simulink model "02_Goniodsky_Mistry_EE547_Project"  (R2018b)
settings: Solver=FixedStepDiscrete  StartTime=0.0  StopTime=inf  RelTol=1e-3  EnableMultiTasking=on
undefined symbols (not defined in the file): DiscIntNeverNeededParam, K, rw
libraries: dspstat3 x2, arduinolib x1, dspsigops x1
settings Model: SimulationMode=external  ExtModeTrigDuration=2  Creator=gonio  LastModifiedBy=GAJJAR
settings OptimizationCC: EnhancedBackFolding=on  PassReuseOutputArgsAs=Individual arguments  MaxStackSize=64  OptimizeBlockOrder=speed  DifferentSizesBufferReuse=on  OptimizationCustomize=off
settings DebuggingCC: ParameterTunabilityLossMsg=error
settings HardwareCC: ProdBitPerInt=16  ProdBitPerPointer=16  ProdBitPerSizeT=16  ProdBitPerPtrDiffT=16  ProdLargestAtomicFloat=None  ProdWordSize=8  ProdHWDeviceType=Atmel->AVR  UseEmbeddedCoderFeatures=off  UseSimulinkCoderFeatures=off
settings SFSimCC: MATLABDynamicMemAlloc=off
settings RTWCC: SystemTargetFile=ert.tlc  HardwareBoard=Arduino Mega 2560  TemplateMakefile=ert_default_tmf  RTWVerbose=off  Toolchain=Arduino AVR  BuildConfiguration=Faster Runs  IncludeHyperlinkInReport=on
settings CodeAppCC: ForceParamTrailComments=on  OperatorAnnotations=on  SimulinkDataObjDesc=on  SFDataObjDesc=on  MangleLength=10  InsertBlockDesc=on
settings ERTTargetCC: SupportContinuousTime=on  SupportNonInlinedSFcns=on  SupportVariableSizeSignals=on  ExtMode=on  ExtModeMexArgs='127.0.0.1' 0 17725  ERTSrcFileBannerTemplate=codertarget_code_template.cgt  ERTHdrFileBannerTemplate=codertarget_code_template.cgt  ERTDataSrcFileTemplate=codertarget_code_template.cgt  ERTDataHdrFileTemplate=codertarget_code_template.cgt

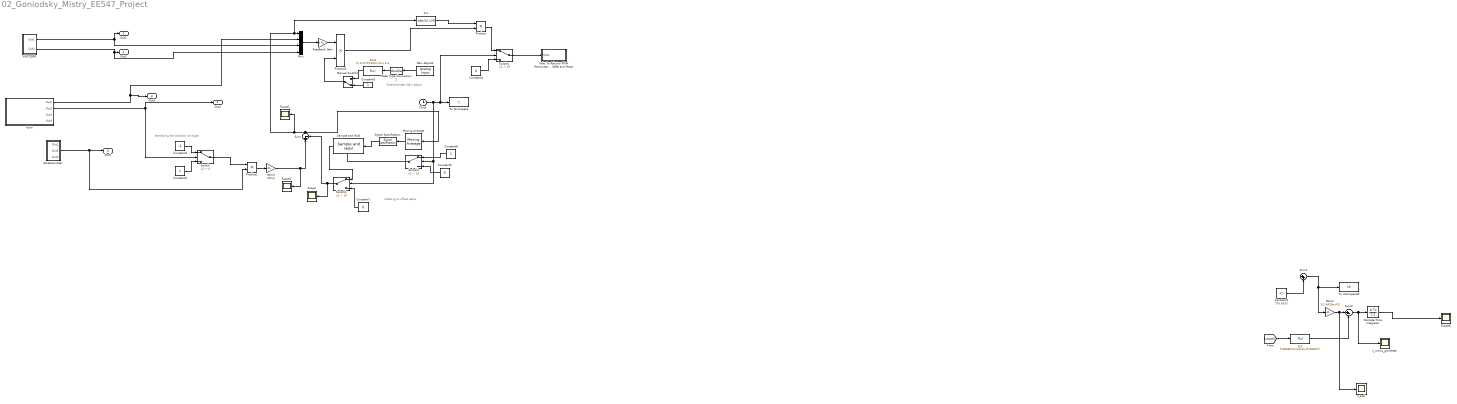
== system 02_Goniodsky_Mistry_EE547_Project ==
  note: Potentiometer Gain Adjust
  note: Identifying the Direction of angle
  note: Intitial gyro offset setup
  Accelerometer : Subsystem
  Clock : Clock
  Constant1 : Constant  Value=376.6633
  Constant2 : Constant
  Constant3 : Constant  Value=-1
  Constant4 : Constant  Value=0
  Constant5 : Constant  Value=0
  Constant6 : Constant
  Constant7 : Constant  Value=0
  Constant9 : Constant
  Data Type Conversion1 : DataTypeConversion  OutDataTypeStr=double
  Discrete-Time Integrator : DiscreteIntegrator  SampleTime=-1  ICPrevOutput=DiscIntNeverNeededParam  ICPrevScaledInput=DiscIntNeverNeededParam
  "ENCODER " : Subsystem
  Fcn : Fcn  Expr=abs(u)<20
  Fcn2 : Fcn  Expr=(1-1/4)*2/1023*u(1)+1/4
  Feedback Gain : Gain  Gain=K  Multiplication=Matrix(K*u)
  Gain Adjust2 : arduinolib/Analog Input  pinNumber=0  ReadResultsOnly=off  ConversionTriggerSource=Software  ExternalTriggerType=uint32(0)  OutputDataType=uint16  EnableConversionCompleteNotify=off  EnableOuputStatus=off  SampleTime=-1  blockPlatform=arduino
  Gain2 : Gain  Gain=1/1.6420e+03
  Gain4 : Gain  Gain=180/pi
  Gyro : Subsystem
  Manual Switch1 : ManualSwitch  CurrentSetting=0
  Moving Average : dspstat3/Moving Average  Method=Sliding window  ForgettingFactorPort=off  SpecifyWindowLength=off  WindowLength=4  ForgettingFactor=0.9  SimulateUsing=Code generation
  Mux : Mux
  Product : Product
  Product1 : Product
  Product2 : Product  RndMeth=Zero
  Sample and Hold : dspsigops/Sample and Hold  trig=Rising edge  initCond=0  latchinput=on
  Scope{,1..2,6} (4 alike) : Scope
  Signal Specification : SignalSpecification  OutDataTypeStr=double  Dimensions=1
  Sum : Sum  Inputs=|+-
  Sum1 : Sum  Inputs=|++
  Sum2 : Sum  Inputs=|+-
  Switch : Switch  Criteria=u2 > Threshold
  Switch1 : Switch  Criteria=u2 > Threshold  Threshold=10
  Switch2 : Switch  Criteria=u2 > Threshold  Threshold=10
  Switch3 : Switch  Criteria=u2 > Threshold  Threshold=10
  To Workspace : ToWorkspace  VariableName=t  SampleTime=-1
  To Workspace3 : ToWorkspace  VariableName=t3  SampleTime=-1
      settings: Save2DSignal=2-D array (concatenate along first dimension)
  Volts To Adruino PWM (NonLinear LOW) 3388 and Motor : Subsystem
  g_z : Fcn  Expr=9.80665*sin(acos(u/9.80665))
  z_acc\ : Scope
  z_minus_gsintheta : Scope
  Out1 : Outport  SignalName=Position
  Out2 : Outport  Port=2  SignalName=Velocity
  Out3 : Outport  Port=3  SignalName=Angular Velocity
  Out4 : Outport  Port=4  SignalName=Angular Position
  Out5 : Outport  Port=5  SignalName=abs_alpha
  wires:
  "ENCODER "/1(Out1) -> Out1/1, Mux/3
  "ENCODER "/2(Out2) -> Mux/4, Out2/1
  Gyro/1(Out1) -> Out3/1, Mux/2
  Gyro/2(Out2) -> Out4/1, Switch/2
  Mux/1 -> Feedback Gain/1
  Fcn/1 -> Product/1
  Clock/1 -> To Workspace/1, Switch1/2, Switch2/2, Switch3/2
  Constant3/1 -> Switch/1
  Constant2/1 -> Switch/3
  Sum1/1 -> Gain2/1, To Workspace3/1
  Gain2/1 -> z_acc\/1, Sum2/1
  Constant1/1 -> Sum1/2
  [yaccel] -> g_z/1
  Sum2/1 -> z_minus_gsintheta/1, Discrete-Time Integrator/1
  g_z/1 -> Sum2/2
  Discrete-Time Integrator/1 -> Scope6/1
  ? -> Sum1/1
  Product1/1 -> Gain4/1
  Accelerometer/2(Out5) -> Out5/1, Product1/2
  Switch/1 -> Product1/1
  Product/1 -> Switch1/1
  Constant4/1 -> Switch1/3
  Switch1/1 -> Volts To Adruino PWM (NonLinear LOW) 3388 and Motor/1(Volts)
  Constant6/1 -> Switch3/1
  Constant5/1 -> Switch3/3
  Switch3/1 -> Sample and Hold/Trigger
  Sample and Hold/1 -> Switch2/1
  Constant7/1 -> Switch2/3
  Switch2/1 -> Scope/1, Sum/2
  Sum/1 -> Scope1/1, Fcn/1, Mux/1, Moving Average/1
  Moving Average/1 -> Signal Specification/1
  Signal Specification/1 -> Sample and Hold/1
  Constant9/1 -> Manual Switch1/2
  Manual Switch1/1 -> Product2/2
  Feedback Gain/1 -> Product2/1
  Product2/1 -> Product/2
  Gain4/1 -> Scope2/1, Sum/1
  Data Type Conversion1/1 -> Fcn2/1
  Gain Adjust2/1 -> Data Type Conversion1/1
  Fcn2/1 -> Manual Switch1/1

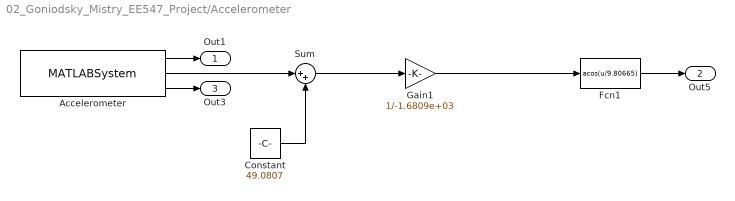
== system 02_Goniodsky_Mistry_EE547_Project/Accelerometer ==
  Accelerometer : MATLABSystem  System=soMPU6050Accel  SimulateUsing=Code generation
      mask Type: soMPU6050Accel
      mask Display:
      | disp('soMPU6050Accel');
      | port_label('output',1,'xaccel');
      | port_label('output',2,'yaccel');
      | port_label('output',3,'zaccel');
  Constant : Constant  Value=49.0807
  Fcn1 : Fcn  Expr=acos(u/9.80665)
  Gain1 : Gain  Gain=1/-1.6809e+03
  Sum : Sum  Inputs=|++
  Out1 : Outport
  Out5 : Outport  Port=2
  Out3 : Outport  Port=3
  wires:
  Gain1/1 -> Fcn1/1
  Accelerometer/3 -> Out3/1
  Fcn1/1 -> Out5/1
  Constant/1 -> Sum/2
  Accelerometer/2 -> Sum/1
  Sum/1 -> Gain1/1
  Accelerometer/1 -> Out1/1

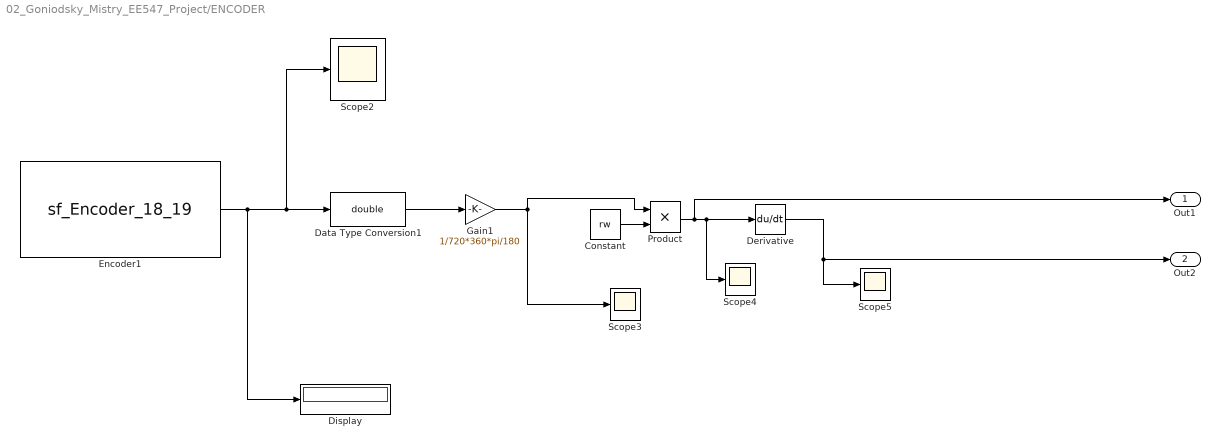
== system 02_Goniodsky_Mistry_EE547_Project/ENCODER  ==
  Constant : Constant  Value=rw
  Data Type Conversion1 : DataTypeConversion  OutDataTypeStr=double
  Derivative : Derivative
  Display : Display
  Encoder1 : S-Function  InitFcn=try, set_param(gcb,'FunctionName','sf_Encoder_18_19'), end  FunctionName=sf_Encoder_18_19  Parameters=uint8(0),uint8(18),uint8(19)  SFunctionModules=sf_Encoder_18_19_wrapper  SFunctionDeploymentMode=off  EnableBusSupport=off  mask(S-Function Builder){}
      mask init:
      | val = [[.9  0.75 0.75 1 1 .9 .9 1]',[1 1 0.75 0.75 .9 .9 1 .9]'];try , sys = get_param(gcb,'SfunBuilderFcnName');if isempty(sys), sys = get_param(gcb,'FunctionName'); end,catch, sys = get_param(gcb,'FunctionName'); end
      settings: CopyFcn=set_param(gcbh,'LinkStatus','none')  PreSaveFcn=try, set_param(gcb,'FunctionName','sf_Encoder_18_19'), end  OpenFcn=sfunctionwizard(gcbh)
      mask Display: plot(val(:,1),val(:,2)),disp(sys), port_label('output',1,'pos')
  Gain1 : Gain  Gain=1/720*360*pi/180
  Product : Product
  Scope{2..5} (4 alike) : Scope
  Out1 : Outport
  Out2 : Outport  Port=2
  wires:
  Gain1/1 -> Product/1, Scope3/1
  Product/1 -> Out1/1, Scope4/1, Derivative/1
  Derivative/1 -> Out2/1, Scope5/1
  Data Type Conversion1/1 -> Gain1/1
  Constant/1 -> Product/2
  Encoder1/1 -> Display/1, Scope2/1, Data Type Conversion1/1

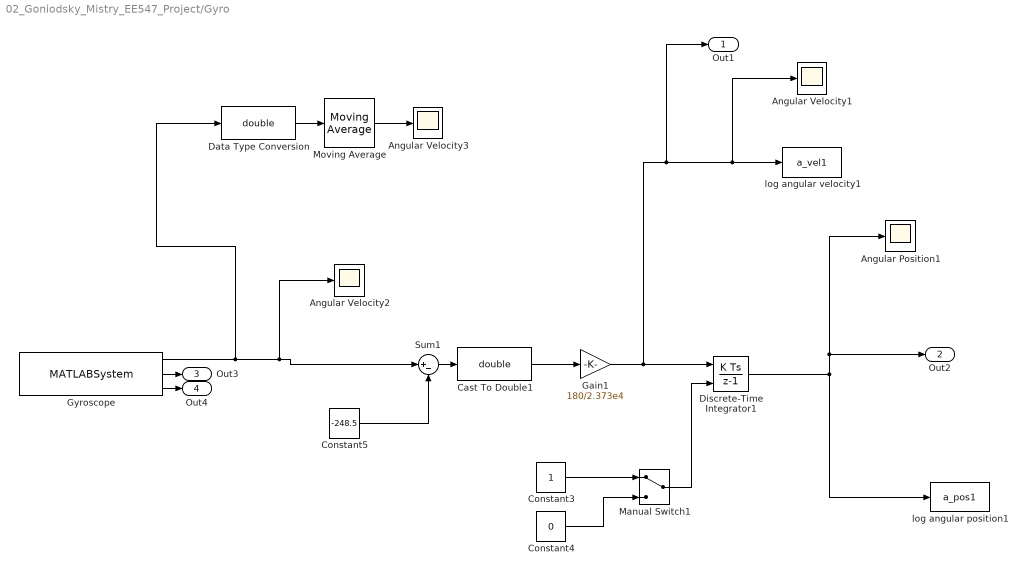
== system 02_Goniodsky_Mistry_EE547_Project/Gyro ==
  Angular Position1 : Scope
  Angular Velocity1 : Scope
  Angular Velocity2 : Scope
  Angular Velocity3 : Scope
  Cast To Double1 : DataTypeConversion  OutDataTypeStr=double
  Constant3 : Constant
  Constant4 : Constant  Value=0
  Constant5 : Constant  Value=-248.5
  Data Type Conversion : DataTypeConversion  OutDataTypeStr=double
  Discrete-Time Integrator1 : DiscreteIntegrator  ExternalReset=either  SampleTime=-1  ICPrevOutput=DiscIntNeverNeededParam  ICPrevScaledInput=DiscIntNeverNeededParam
  Gain1 : Gain  Gain=180/2.373e4
  Gyroscope : MATLABSystem  System=soMPU6050Gyro  DLPFmode=0
      mask Type: soMPU6050Gyro
      mask Display:
      | disp('soMPU6050Gyro');
      | port_label('output',1,'xvel');
      | port_label('output',2,'yvel');
      | port_label('output',3,'zvel');
  Manual Switch1 : ManualSwitch
  Moving Average : dspstat3/Moving Average  Method=Sliding window  ForgettingFactorPort=off  SpecifyWindowLength=on  WindowLength=200  ForgettingFactor=0.9  SimulateUsing=Code generation
  Sum1 : Sum  Inputs=|+-
  log angular position1 : ToWorkspace  VariableName=a_pos1  SampleTime=-1
  log angular velocity1 : ToWorkspace  VariableName=a_vel1  SampleTime=-1
  Out1 : Outport
  Out2 : Outport  Port=2
  Out3 : Outport  Port=3
  Out4 : Outport  Port=4
  wires:
  Discrete-Time Integrator1/1 -> log angular position1/1, Out2/1, Angular Position1/1
  Gyroscope/1 -> Data Type Conversion/1, Angular Velocity2/1, Sum1/1
  Sum1/1 -> Cast To Double1/1
  Gain1/1 -> Out1/1, Angular Velocity1/1, log angular velocity1/1, Discrete-Time Integrator1/1
  Constant3/1 -> Manual Switch1/1
  Constant4/1 -> Manual Switch1/2
  Manual Switch1/1 -> Discrete-Time Integrator1/2
  Cast To Double1/1 -> Gain1/1
  Constant5/1 -> Sum1/2
  Moving Average/1 -> Angular Velocity3/1
  Gyroscope/2 -> Out3/1
  Data Type Conversion/1 -> Moving Average/1
  Gyroscope/3 -> Out4/1

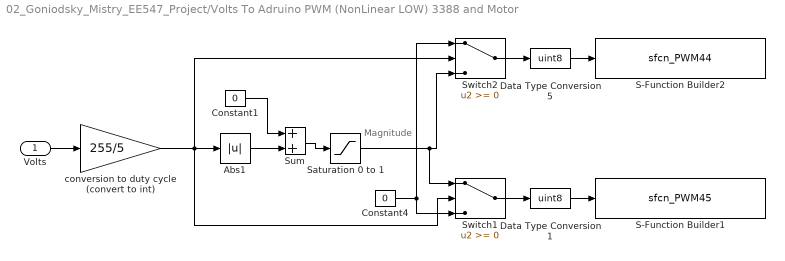
== system 02_Goniodsky_Mistry_EE547_Project/Volts To Adruino PWM (NonLinear LOW) 3388 and Motor ==
  note: Magnitude
  Volts : Inport
  Abs1 : Abs
  Constant1 : Constant  Value=0
  Constant4 : Constant  Value=0
  Data Type Conversion1 : DataTypeConversion  OutDataTypeStr=uint8
  Data Type Conversion5 : DataTypeConversion  OutDataTypeStr=uint8
  S-Function Builder1 : S-Function  InitFcn=try, set_param(gcb,'FunctionName','sfcn_PWM45'), end  FunctionName=sfcn_PWM45  Parameters=uint8(5)  SFunctionModules=sfcn_PWM45_wrapper  SFunctionDeploymentMode=off  EnableBusSupport=off  mask(S-Function Builder){}
      mask init: same as 02_Goniodsky_Mistry_EE547_Project/ENCODER /Encoder1
      settings: CopyFcn=set_param(gcbh,'LinkStatus','none')  PreSaveFcn=try, set_param(gcb,'FunctionName','sfcn_PWM45'), end  OpenFcn=sfunctionwizard(gcbh)
      mask Display: plot(val(:,1),val(:,2)),disp(sys), port_label('input',1,'in')
  S-Function Builder2 : S-Function  InitFcn=try, set_param(gcb,'FunctionName','sfcn_PWM44'), end  FunctionName=sfcn_PWM44  Parameters=uint8(2)  SFunctionModules=sfcn_PWM44_wrapper  SFunctionDeploymentMode=off  EnableBusSupport=off  mask(S-Function Builder){}
      mask init: same as 02_Goniodsky_Mistry_EE547_Project/ENCODER /Encoder1
      settings: CopyFcn=set_param(gcbh,'LinkStatus','none')  PreSaveFcn=try, set_param(gcb,'FunctionName','sfcn_PWM44'), end  OpenFcn=sfunctionwizard(gcbh)
      mask Display: plot(val(:,1),val(:,2)),disp(sys), port_label('input',1,'in')
  Saturation 0 to 1 : Saturate  UpperLimit=255  LowerLimit=0
  Sum : Sum
  Switch1 : Switch
  Switch2 : Switch
  conversion to duty cycle (convert to int) : Gain  Gain=255/5  OutDataTypeStr=int16
  wires:
  Volts/1 -> conversion to duty cycle (convert to int)/1
  conversion to duty cycle (convert to int)/1 -> Switch1/2, Abs1/1, Switch2/2
  Switch2/1 -> Data Type Conversion5/1
  Switch1/1 -> Data Type Conversion1/1
  Data Type Conversion5/1 -> S-Function Builder2/1
  Data Type Conversion1/1 -> S-Function Builder1/1
  Abs1/1 -> Sum/2
  Sum/1 -> Saturation 0 to 1/1
  Constant1/1 -> Sum/1
  Constant4/1 -> Switch2/1, Switch1/3
  Saturation 0 to 1/1 -> Switch2/3, Switch1/1
